simulink model "MFunctionBus"  (R2017b)
settings: Solver=FixedStepDiscrete  StartTime=0.0  StopTime=1  FixedStep=1.000000  RelTol=1e-3  EnableMultiTasking=on
PreLoadFcn:
  | load businfo.mat;
settings Model: Creator=The MathWorks, Inc.  LastModifiedBy=hbourbou
settings DataIOCC: LimitDataPoints=on  SaveFormat=Array
settings OptimizationCC: ExpressionDepthLimit=2147483647  InitFltsAndDblsToZero=on  LifeSpan=inf
settings DebuggingCC: SaveWithParameterizedLinksMsg=none  UnderspecifiedInitializationDetection=Classic  MergeDetectMultiDrivingBlocksExec=none  SignalResolutionControl=TryResolveAllWithWarning  SolverPrmCheckMsg=warning  FcnCallInpInsideContextMsg=warning  StateNameClashWarn=warning  SFUnexpectedBacktrackingDiag=warning  SFNoUnconditionalDefaultTransitionDiag=warning  SFExecutionAtInitializationDiag=none
settings HardwareCC: ProdBitPerPointer=32  ProdBitPerSizeT=32  ProdBitPerPtrDiffT=32  ProdLargestAtomicFloat=None  ProdIntDivRoundTo=Undefined  ProdEndianess=Unspecified  ProdWordSize=32  ProdHWDeviceType=32-bit Generic
settings ModelReferenceCC: PropagateSignalLabelsOutOfModel=off
settings SFSimCC: SimParseCustomCode=off
settings CodeAppCC: StateflowObjectComments=on
settings GRTTargetCC: TargetFcnLib=ansi_tfl_tmw.mat  TargetLangStandard=C89/C90 (ANSI)  GeneratePreprocessorConditionals=Disable all  CombineOutputUpdateFcns=off  GRTInterface=on
settings ConfigComp: CovMetricSettings=dw  CovHtmlReporting=on  CovSaveCumulativeToWorkspaceVar=on  CovSaveSingleToWorkspaceVar=on  CovExternalEMLEnable=off  CovSFcnEnable=off

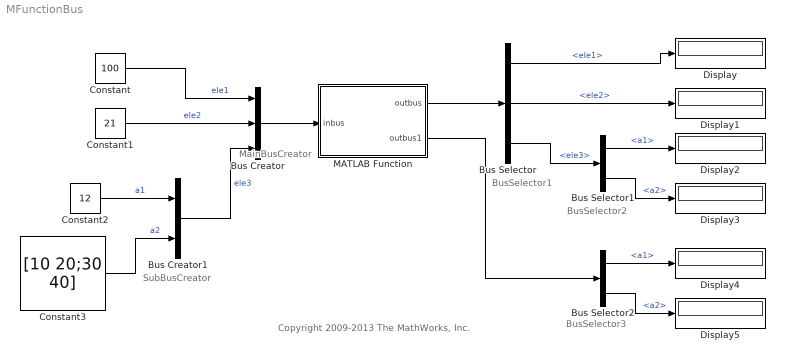
== system MFunctionBus ==
  note: BusSelector1
  note: SubBusCreator
  note: MainBusCreator
  note: BusSelector2
  note: BusSelector3
  note: Copyright 2009-2013 The MathWorks, Inc.
  Bus Creator : BusCreator  Inputs=3  OutDataTypeStr=Bus: MainBus  NonVirtualBus=on
  Bus Creator1 : BusCreator  Inputs=2  OutDataTypeStr=Bus: SubBus  NonVirtualBus=on
  Bus Selector : BusSelector  OutputSignals=ele1,ele2,ele3
  Bus Selector1 : BusSelector  OutputSignals=a1,a2
  Bus Selector2 : BusSelector  OutputSignals=a1,a2
  Constant : Constant  Value=100  OutDataTypeStr=double
  Constant1 : Constant  Value=21  OutDataTypeStr=single
  Constant2 : Constant  Value=12  OutDataTypeStr=double
  Constant3 : Constant  Value=[10 20;30 40]  OutDataTypeStr=int8
  Display{,1..5} (6 alike) : Display
  MATLAB Function : MATLAB Function  TreatAsAtomicUnit=on
  wires:
  Constant/1 -> Bus Creator/1  "ele1"
  Constant1/1 -> Bus Creator/2  "ele2"
  Bus Creator1/1 -> Bus Creator/3  "ele3"
  Constant2/1 -> Bus Creator1/1  "a1"
  Constant3/1 -> Bus Creator1/2  "a2"
  Bus Creator/1 -> MATLAB Function/1(inbus)
  MATLAB Function/1(outbus) -> Bus Selector/1
  Bus Selector/1 -> Display/1  "<ele1>"
  Bus Selector/2 -> Display1/1  "<ele2>"
  Bus Selector/3 -> Bus Selector1/1  "<ele3>"
  Bus Selector1/1 -> Display2/1  "<a1>"
  Bus Selector1/2 -> Display3/1  "<a2>"
  Bus Selector2/1 -> Display4/1  "<a1>"
  Bus Selector2/2 -> Display5/1  "<a2>"
  MATLAB Function/2(outbus1) -> Bus Selector2/1

== matlab function MFunctionBus/MATLAB Function ==
  data: inbus input; outbus output Bus: MainBus size=1; outbus1 output Bus: SubBus size=1
function [outbus, outbus1] = fcn(inbus)
%#codegen

substruct.a1 = inbus.ele3.a1;
substruct.a2 = int8([1 2;3 4]);

mystruct = struct('ele1',20.5, 'ele2', single(100), 'ele3', substruct);

outbus = mystruct;
outbus.ele3.a2 = 2*(substruct.a2);

outbus1 = inbus.ele3;
